simulink model "FaultCheck"  (R2022b)
settings: Solver=FixedStepAuto  StartTime=0.0  StopTime=10  FixedStep=1  RelTol=1e-3
undefined symbols (not defined in the file): C_Flt_IGBTULowerTempConfirmTh_u16, C_Flt_IGBTULowerTempDiagEn_b, C_Flt_IGBTULowerTempErrCode_u16, C_Flt_IGBTULowerTempPowerCoeff, C_Flt_IGBTULowerTempRecoveryTh_u16, C_Flt_IGBTULowerTempRecTh_s32, C_Flt_IGBTULowerTempTrigTh_s32, C_Flt_IGBTUOverTempConfirmTh_u16, C_Flt_IGBTUOverTempDiagEn_b, C_Flt_IGBTUOverTempErrCode_u16, C_Flt_IGBTUOverTempRecoveryTh_u16, C_Flt_IGBTUOverTempRecTh_s32, C_Flt_IGBTUOverTempTrigTh_s32, C_Flt_IGBTVLowerTempConfirmTh_u16, C_Flt_IGBTVLowerTempDiagEn_b, C_Flt_IGBTVLowerTempErrCode_u16, C_Flt_IGBTVLowerTempPowerCoeff, C_Flt_IGBTVLowerTempRecoveryTh_u16, C_Flt_IGBTVLowerTempRecTh_s32, C_Flt_IGBTVLowerTempTrigTh_s32, C_Flt_IGBTVOverTempConfirmTh_u16, C_Flt_IGBTVOverTempDiagEn_b, C_Flt_IGBTVOverTempErrCode_u16, C_Flt_IGBTVOverTempRecoveryTh_u16, C_Flt_IGBTVOverTempRecTh_s32, C_Flt_IGBTVOverTempTrigTh_s32, C_Flt_IGBTWLowerTempConfirmTh_u16, C_Flt_IGBTWLowerTempDiagEn_b, C_Flt_IGBTWLowerTempErrCode_u16, C_Flt_IGBTWLowerTempPowerCoeff, C_Flt_IGBTWLowerTempRecoveryTh_u16, C_Flt_IGBTWLowerTempRecTh_s32, C_Flt_IGBTWLowerTempTrigTh_s32, C_Flt_IGBTWOverTempConfirmTh_u16, C_Flt_IGBTWOverTempDiagEn_b, C_Flt_IGBTWOverTempErrCode_u16, C_Flt_IGBTWOverTempRecoveryTh_u16, C_Flt_IGBTWOverTempRecTh_s32, C_Flt_IGBTWOverTempTrigTh_s32, C_Flt_IuOCConfirmTh_u16, C_Flt_IuOCDiagEn_b, C_Flt_IuOCErrCode_u16, C_Flt_IuOCNegLimit_s32, C_Flt_IuOCPosLimit_s32, C_Flt_IuOCRecoveryTh_u16, C_Flt_IuZeroDriftDiagEn_b, C_Flt_IuZeroDriftErrCode_u16, C_Flt_IvOCConfirmTh_u16, C_Flt_IvOCDiagEn_b, C_Flt_IvOCErrCode_u16, C_Flt_IvOCNegLimit_s32, C_Flt_IvOCPosLimit_s32, C_Flt_IvOCRecoveryTh_u16, C_Flt_IvZeroDriftDiagEn_b, C_Flt_IvZeroDriftErrCode_u16, C_Flt_IwOCConfirmTh_u16, C_Flt_IwOCDiagEn_b, C_Flt_IwOCErrCode_u16, C_Flt_IwOCNegLimit_s32, C_Flt_IwOCPosLimit_s32 ... (+196)
libraries: YS_UserDefined_Library x21, simulink x5
(part 8 of 11)

== system FaultCheck/FaultDiagnose/IGBTTempDiag/IGBTVLowerTempDiag/Diagnose/NormalDiag ==
  IGBTVTemp : Inport
  Parameter : Inport  Port=2
  Action Port : ActionPort  ActionPortLabel=else
  Bus Selector : BusSelector  OutputSignals=IGBTVLowerTempConfirmTh,IGBTVLowerTempRecoveryTh,IGBTVLowerTempTrigTh,IGBTVLowerTempRecTh
  DebounceRecInTwo : YS_UserDefined_Library/Fault/DebounceRecInTwo  SystemSampleTime=-1  VariantActivationTime=update diagram  Latency=0  AutoFrameSizeCalculation=off
      settings: SourceProductName=YS
  Relational Operator : RelationalOperator  Operator=>  OutDataTypeStr=boolean  RndMeth=Simplest  InputSameDT=off
  Relational Operator1 : RelationalOperator  Operator=>  OutDataTypeStr=boolean  RndMeth=Simplest  InputSameDT=off
  Signal Copy : SignalConversion  OverrideOpt=off
  IGBTVLowerTempFltDeb : Outport
  wires:
  Parameter/1 -> Bus Selector/1
  Bus Selector/1 -> DebounceRecInTwo/1  "<IGBTVLowerTempConfirmTh>"
  Bus Selector/2 -> DebounceRecInTwo/2  "<IGBTVLowerTempRecoveryTh>"
  DebounceRecInTwo/1 -> Signal Copy/1  "M_Flt_IGBTVLowerTempFltFlgDeb_b"
  Relational Operator/1 -> DebounceRecInTwo/3  "M_Flt_IGBTVLowerTempFltFlgUnDeb_b"
  Signal Copy/1 -> IGBTVLowerTempFltDeb/1
  Bus Selector/3 -> Relational Operator/1  "<IGBTVLowerTempTrigTh>"
  IGBTVTemp/1 -> Relational Operator1/1, Relational Operator/2
  Bus Selector/4 -> Relational Operator1/2  "<IGBTVLowerTempRecTh>"
  Relational Operator1/1 -> DebounceRecInTwo/4  "M_Flt_IGBTVLowerTempRecFlgUnDeb_b"

== system FaultCheck/FaultDiagnose/IGBTTempDiag/IGBTVLowerTempDiag/FaultLevelDeter/LowerOne ==
  FaultLevel : Inport
  Action Port : ActionPort  ActionPortLabel=else
  IGBTVLowerTempFltLevel : Outport
  wires:
  FaultLevel/1 -> IGBTVLowerTempFltLevel/1

== system FaultCheck/FaultDiagnose/IGBTTempDiag/IGBTVLowerTempDiag/FaultLevelDeter/Normal ==
  Action Port : ActionPort  ActionPortLabel=if(u1 == 0)
  Constant : Constant  Value=C_Flt_LevelZero_u8
  IGBTVLowerTempFltLevel : Outport
  wires:
  Constant/1 -> IGBTVLowerTempFltLevel/1

== system FaultCheck/FaultDiagnose/IGBTTempDiag/IGBTVLowerTempDiag/PowerReductionCoeffDeter/If Action Subsystem ==
  Action Port : ActionPort  ActionPortLabel=if(u1 < 2)
  Constant : Constant  Value=C_Flt_PowerCoeffOne_s32
  Coeff : Outport
  wires:
  Constant/1 -> Coeff/1

== system FaultCheck/FaultDiagnose/IGBTTempDiag/IGBTVLowerTempDiag/PowerReductionCoeffDeter/If Action Subsystem1 ==
  PowerCoeff : Inport
  Action Port : ActionPort  ActionPortLabel=elseif(u1 == 2)
  Coeff : Outport
  wires:
  PowerCoeff/1 -> Coeff/1

== system FaultCheck/FaultDiagnose/IGBTTempDiag/IGBTVLowerTempDiag/PowerReductionCoeffDeter/If Action Subsystem2 ==
  Action Port : ActionPort  ActionPortLabel=else
  Constant : Constant  Value=C_Flt_PowerCoeffZero_s32
  Coeff : Outport
  wires:
  Constant/1 -> Coeff/1

== system FaultCheck/FaultDiagnose/IGBTTempDiag/IGBTVOverTempDiag/Diagnose/Disable ==
  Action Port : ActionPort  ActionPortLabel=if(u1 == 0)
  Constant : Constant  Value=C_Flt_NoErr_b
  IGBTVOverTempFltDeb : Outport
  wires:
  Constant/1 -> IGBTVOverTempFltDeb/1

== system FaultCheck/FaultDiagnose/IGBTTempDiag/IGBTVOverTempDiag/Diagnose/NormalDiag ==
  IGBTVTemp : Inport
  Parameter : Inport  Port=2
  Action Port : ActionPort  ActionPortLabel=else
  Bus Selector : BusSelector  OutputSignals=IGBTVOverTempConfirmTh,IGBTVOverTempRecoveryTh,IGBTVOverTempTrigTh,IGBTVOverTempRecTh
  DebounceRecInTwo : YS_UserDefined_Library/Fault/DebounceRecInTwo  SystemSampleTime=-1  VariantActivationTime=update diagram  Latency=0  AutoFrameSizeCalculation=off
      settings: SourceProductName=YS
  Relational Operator : RelationalOperator  Operator=<  OutDataTypeStr=boolean  RndMeth=Simplest  InputSameDT=off
  Relational Operator1 : RelationalOperator  Operator=<  OutDataTypeStr=boolean  RndMeth=Simplest  InputSameDT=off
  Signal Copy : SignalConversion  OverrideOpt=off
  IGBTVOverTempFltDeb : Outport
  wires:
  Relational Operator1/1 -> DebounceRecInTwo/4  "M_Flt_IGBTVOverTempRecFlgUnDeb_b"
  Bus Selector/4 -> Relational Operator1/2  "<IGBTVOverTempRecTh>"
  IGBTVTemp/1 -> Relational Operator1/1, Relational Operator/2
  Bus Selector/3 -> Relational Operator/1  "<IGBTVOverTempTrigTh>"
  Signal Copy/1 -> IGBTVOverTempFltDeb/1
  Relational Operator/1 -> DebounceRecInTwo/3  "M_Flt_IGBTVOverTempFltFlgUnDeb_b"
  DebounceRecInTwo/1 -> Signal Copy/1  "M_Flt_IGBTVOverTempFltFlgDeb_b"
  Bus Selector/2 -> DebounceRecInTwo/2  "<IGBTVOverTempRecoveryTh>"
  Bus Selector/1 -> DebounceRecInTwo/1  "<IGBTVOverTempConfirmTh>"
  Parameter/1 -> Bus Selector/1

== system FaultCheck/FaultDiagnose/IGBTTempDiag/IGBTVOverTempDiag/FaultLevelDeter/LowerOne ==
  FaultLevel : Inport
  Action Port : ActionPort  ActionPortLabel=else
  IGBTVOverTempFltLevel : Outport
  wires:
  FaultLevel/1 -> IGBTVOverTempFltLevel/1

== system FaultCheck/FaultDiagnose/IGBTTempDiag/IGBTVOverTempDiag/FaultLevelDeter/Normal ==
  Action Port : ActionPort  ActionPortLabel=if(u1 == 0)
  Constant : Constant  Value=C_Flt_LevelZero_u8
  IGBTVOverTempFltLevel : Outport
  wires:
  Constant/1 -> IGBTVOverTempFltLevel/1

== system FaultCheck/FaultDiagnose/IGBTTempDiag/IGBTVOverTempDiag/PowerReductionCoeffDeter/If Action Subsystem ==
  Action Port : ActionPort  ActionPortLabel=if(u1 < 2)
  Constant : Constant  Value=C_Flt_PowerCoeffOne_s32
  Coeff : Outport
  wires:
  Constant/1 -> Coeff/1

== system FaultCheck/FaultDiagnose/IGBTTempDiag/IGBTVOverTempDiag/PowerReductionCoeffDeter/If Action Subsystem1 ==
  PowerCoeff : Inport
  Action Port : ActionPort  ActionPortLabel=elseif(u1 == 2)
  Coeff : Outport
  wires:
  PowerCoeff/1 -> Coeff/1

== system FaultCheck/FaultDiagnose/IGBTTempDiag/IGBTVOverTempDiag/PowerReductionCoeffDeter/If Action Subsystem2 ==
  Action Port : ActionPort  ActionPortLabel=else
  Constant : Constant  Value=C_Flt_PowerCoeffZero_s32
  Coeff : Outport
  wires:
  Constant/1 -> Coeff/1

== system FaultCheck/FaultDiagnose/IGBTTempDiag/IGBTWLowerTempDiag/Diagnose/Disable ==
  Action Port : ActionPort  ActionPortLabel=if(u1 == 0)
  Constant : Constant  Value=C_Flt_NoErr_b
  IGBTWLowerTempFltDeb : Outport
  wires:
  Constant/1 -> IGBTWLowerTempFltDeb/1

== system FaultCheck/FaultDiagnose/IGBTTempDiag/IGBTWLowerTempDiag/Diagnose/NormalDiag ==
  IGBTWTemp : Inport
  Parameter : Inport  Port=2
  Action Port : ActionPort  ActionPortLabel=else
  Bus Selector : BusSelector  OutputSignals=IGBTWLowerTempConfirmTh,IGBTWLowerTempRecoveryTh,IGBTWLowerTempTrigTh,IGBTWLowerTempRecTh
  DebounceRecInTwo : YS_UserDefined_Library/Fault/DebounceRecInTwo  SystemSampleTime=-1  VariantActivationTime=update diagram  Latency=0  AutoFrameSizeCalculation=off
      settings: SourceProductName=YS
  Relational Operator : RelationalOperator  Operator=>  OutDataTypeStr=boolean  RndMeth=Simplest  InputSameDT=off
  Relational Operator1 : RelationalOperator  Operator=>  OutDataTypeStr=boolean  RndMeth=Simplest  InputSameDT=off
  Signal Copy : SignalConversion  OverrideOpt=off
  IGBTWLowerTempFltDeb : Outport
  wires:
  Parameter/1 -> Bus Selector/1
  Bus Selector/1 -> DebounceRecInTwo/1  "<IGBTWLowerTempConfirmTh>"
  Bus Selector/2 -> DebounceRecInTwo/2  "<IGBTWLowerTempRecoveryTh>"
  DebounceRecInTwo/1 -> Signal Copy/1  "M_Flt_IGBTWLowerTempFltFlgDeb_b"
  Relational Operator/1 -> DebounceRecInTwo/3  "M_Flt_IGBTWLowerTempFltFlgUnDeb_b"
  Signal Copy/1 -> IGBTWLowerTempFltDeb/1
  Bus Selector/3 -> Relational Operator/1  "<IGBTWLowerTempTrigTh>"
  IGBTWTemp/1 -> Relational Operator1/1, Relational Operator/2
  Bus Selector/4 -> Relational Operator1/2  "<IGBTWLowerTempRecTh>"
  Relational Operator1/1 -> DebounceRecInTwo/4  "M_Flt_IGBTWLowerTempRecFlgUnDeb_b"

== system FaultCheck/FaultDiagnose/IGBTTempDiag/IGBTWLowerTempDiag/FaultLevelDeter/LowerOne ==
  FaultLevel : Inport
  Action Port : ActionPort  ActionPortLabel=else
  IGBTWLowerTempFltLevel : Outport
  wires:
  FaultLevel/1 -> IGBTWLowerTempFltLevel/1

== system FaultCheck/FaultDiagnose/IGBTTempDiag/IGBTWLowerTempDiag/FaultLevelDeter/Normal ==
  Action Port : ActionPort  ActionPortLabel=if(u1 == 0)
  Constant : Constant  Value=C_Flt_LevelZero_u8
  IGBTWLowerTempFltLevel : Outport
  wires:
  Constant/1 -> IGBTWLowerTempFltLevel/1

== system FaultCheck/FaultDiagnose/IGBTTempDiag/IGBTWLowerTempDiag/PowerReductionCoeffDeter/If Action Subsystem ==
  Action Port : ActionPort  ActionPortLabel=if(u1 < 2)
  Constant : Constant  Value=C_Flt_PowerCoeffOne_s32
  Coeff : Outport
  wires:
  Constant/1 -> Coeff/1

== system FaultCheck/FaultDiagnose/IGBTTempDiag/IGBTWLowerTempDiag/PowerReductionCoeffDeter/If Action Subsystem1 ==
  PowerCoeff : Inport
  Action Port : ActionPort  ActionPortLabel=elseif(u1 == 2)
  Coeff : Outport
  wires:
  PowerCoeff/1 -> Coeff/1

== system FaultCheck/FaultDiagnose/IGBTTempDiag/IGBTWLowerTempDiag/PowerReductionCoeffDeter/If Action Subsystem2 ==
  Action Port : ActionPort  ActionPortLabel=else
  Constant : Constant  Value=C_Flt_PowerCoeffZero_s32
  Coeff : Outport
  wires:
  Constant/1 -> Coeff/1

== system FaultCheck/FaultDiagnose/IGBTTempDiag/IGBTWOverTempDiag/Diagnose/Disable ==
  Action Port : ActionPort  ActionPortLabel=if(u1 == 0)
  Constant : Constant  Value=C_Flt_NoErr_b
  IGBTWOverTempFltDeb : Outport
  wires:
  Constant/1 -> IGBTWOverTempFltDeb/1

== system FaultCheck/FaultDiagnose/IGBTTempDiag/IGBTWOverTempDiag/Diagnose/NormalDiag ==
  IGBTWTemp : Inport
  Parameter : Inport  Port=2
  Action Port : ActionPort  ActionPortLabel=else
  Bus Selector : BusSelector  OutputSignals=IGBTWOverTempConfirmTh,IGBTWOverTempRecoveryTh,IGBTWOverTempTrigTh,IGBTWOverTempRecTh
  DebounceRecInTwo : YS_UserDefined_Library/Fault/DebounceRecInTwo  SystemSampleTime=-1  VariantActivationTime=update diagram  Latency=0  AutoFrameSizeCalculation=off
      settings: SourceProductName=YS
  Relational Operator : RelationalOperator  Operator=<  OutDataTypeStr=boolean  RndMeth=Simplest  InputSameDT=off
  Relational Operator1 : RelationalOperator  Operator=<  OutDataTypeStr=boolean  RndMeth=Simplest  InputSameDT=off
  Signal Copy : SignalConversion  OverrideOpt=off
  IGBTWOverTempFltDeb : Outport
  wires:
  Parameter/1 -> Bus Selector/1
  Bus Selector/1 -> DebounceRecInTwo/1  "<IGBTWOverTempConfirmTh>"
  Bus Selector/2 -> DebounceRecInTwo/2  "<IGBTWOverTempRecoveryTh>"
  DebounceRecInTwo/1 -> Signal Copy/1  "M_Flt_IGBTWOverTempFltFlgDeb_b"
  Relational Operator/1 -> DebounceRecInTwo/3  "M_Flt_IGBTWOverTempFltFlgUnDeb_b"
  Signal Copy/1 -> IGBTWOverTempFltDeb/1
  Bus Selector/3 -> Relational Operator/1  "<IGBTWOverTempTrigTh>"
  IGBTWTemp/1 -> Relational Operator1/1, Relational Operator/2
  Bus Selector/4 -> Relational Operator1/2  "<IGBTWOverTempRecTh>"
  Relational Operator1/1 -> DebounceRecInTwo/4  "M_Flt_IGBTWOverTempRecFlgUnDeb_b"

== system FaultCheck/FaultDiagnose/IGBTTempDiag/IGBTWOverTempDiag/FaultLevelDeter/LowerOne ==
  FaultLevel : Inport
  Action Port : ActionPort  ActionPortLabel=else
  IGBTWOverTempFltLevel : Outport
  wires:
  FaultLevel/1 -> IGBTWOverTempFltLevel/1

== system FaultCheck/FaultDiagnose/IGBTTempDiag/IGBTWOverTempDiag/FaultLevelDeter/Normal ==
  Action Port : ActionPort  ActionPortLabel=if(u1 == 0)
  Constant : Constant  Value=C_Flt_LevelZero_u8
  IGBTWOverTempFltLevel : Outport
  wires:
  Constant/1 -> IGBTWOverTempFltLevel/1

== system FaultCheck/FaultDiagnose/IGBTTempDiag/IGBTWOverTempDiag/PowerReductionCoeffDeter/If Action Subsystem ==
  Action Port : ActionPort  ActionPortLabel=if(u1 < 2)
  Constant : Constant  Value=C_Flt_PowerCoeffOne_s32
  Coeff : Outport
  wires:
  Constant/1 -> Coeff/1

== system FaultCheck/FaultDiagnose/IGBTTempDiag/IGBTWOverTempDiag/PowerReductionCoeffDeter/If Action Subsystem1 ==
  PowerCoeff : Inport
  Action Port : ActionPort  ActionPortLabel=elseif(u1 == 2)
  Coeff : Outport
  wires:
  PowerCoeff/1 -> Coeff/1

== system FaultCheck/FaultDiagnose/IGBTTempDiag/IGBTWOverTempDiag/PowerReductionCoeffDeter/If Action Subsystem2 ==
  Action Port : ActionPort  ActionPortLabel=else
  Constant : Constant  Value=C_Flt_PowerCoeffZero_s32
  Coeff : Outport
  wires:
  Constant/1 -> Coeff/1

== system FaultCheck/FaultDiagnose/MotorSpdFltDiag/MotorOverSpdOneNegDiag/Diagnose/Disable ==
  Action Port : ActionPort  ActionPortLabel=if(u1 == 0)
  Constant : Constant  Value=C_Flt_NoErr_b
  MotorOverSpdOneNegFltDeb : Outport
  wires:
  Constant/1 -> MotorOverSpdOneNegFltDeb/1

== system FaultCheck/FaultDiagnose/MotorSpdFltDiag/MotorOverSpdOneNegDiag/Diagnose/NormalDiag ==
  MotorSpd : Inport
  Parameter : Inport  Port=2
  Action Port : ActionPort  ActionPortLabel=else
  Bus Selector : BusSelector  OutputSignals=MotorOverSpdOneNegConfirmTh,MotorOverSpdOneNegRecoveryTh,MotorOverSpdOneNegTrigTh,MotorOverSpdOneNegRecTh
  DebounceRecInTwo : YS_UserDefined_Library/Fault/DebounceRecInTwo  SystemSampleTime=-1  VariantActivationTime=update diagram  Latency=0  AutoFrameSizeCalculation=off
      settings: SourceProductName=YS
  Relational Operator : RelationalOperator  Operator=>  OutDataTypeStr=boolean  RndMeth=Simplest  InputSameDT=off
  Relational Operator1 : RelationalOperator  Operator=>  OutDataTypeStr=boolean  RndMeth=Simplest  InputSameDT=off
  Signal Copy : SignalConversion  OverrideOpt=off
  MotorOverSpdOneNegFltDeb : Outport
  wires:
  Parameter/1 -> Bus Selector/1
  Bus Selector/1 -> DebounceRecInTwo/1  "<MotorOverSpdOneNegConfirmTh>"
  Bus Selector/2 -> DebounceRecInTwo/2  "<MotorOverSpdOneNegRecoveryTh>"
  DebounceRecInTwo/1 -> Signal Copy/1  "M_Flt_MotorOverSpdOneNegFltFlgDeb_b"
  Relational Operator/1 -> DebounceRecInTwo/3  "M_Flt_MotorOverSpdOneNegFltFlgUnDeb_b"
  Signal Copy/1 -> MotorOverSpdOneNegFltDeb/1
  Bus Selector/3 -> Relational Operator/1  "<MotorOverSpdOneNegTrigTh>"
  MotorSpd/1 -> Relational Operator1/1, Relational Operator/2
  Bus Selector/4 -> Relational Operator1/2  "<MotorOverSpdOneNegRecTh>"
  Relational Operator1/1 -> DebounceRecInTwo/4  "M_Flt_MotorOverSpdOneNegRecFlgUnDeb_b"

== system FaultCheck/FaultDiagnose/MotorSpdFltDiag/MotorOverSpdOneNegDiag/FaultLevelDeter/LowerOne ==
  FaultLevel : Inport
  Action Port : ActionPort  ActionPortLabel=else
  MotorOverSpdOneNegFltLevel : Outport
  wires:
  FaultLevel/1 -> MotorOverSpdOneNegFltLevel/1

== system FaultCheck/FaultDiagnose/MotorSpdFltDiag/MotorOverSpdOneNegDiag/FaultLevelDeter/Normal ==
  Action Port : ActionPort  ActionPortLabel=if(u1 == 0)
  Constant : Constant  Value=C_Flt_LevelZero_u8
  MotorOverSpdOneNegFltLevel : Outport
  wires:
  Constant/1 -> MotorOverSpdOneNegFltLevel/1

== system FaultCheck/FaultDiagnose/MotorSpdFltDiag/MotorOverSpdOneNegDiag/PowerReductionCoeffDeter/If Action Subsystem ==
  Action Port : ActionPort  ActionPortLabel=if(u1 < 2)
  Constant : Constant  Value=C_Flt_PowerCoeffOne_s32
  Coeff : Outport
  wires:
  Constant/1 -> Coeff/1

== system FaultCheck/FaultDiagnose/MotorSpdFltDiag/MotorOverSpdOneNegDiag/PowerReductionCoeffDeter/If Action Subsystem1 ==
  PowerCoeff : Inport
  Action Port : ActionPort  ActionPortLabel=elseif(u1 == 2)
  Coeff : Outport
  wires:
  PowerCoeff/1 -> Coeff/1

== system FaultCheck/FaultDiagnose/MotorSpdFltDiag/MotorOverSpdOneNegDiag/PowerReductionCoeffDeter/If Action Subsystem2 ==
  Action Port : ActionPort  ActionPortLabel=else
  Constant : Constant  Value=C_Flt_PowerCoeffZero_s32
  Coeff : Outport
  wires:
  Constant/1 -> Coeff/1

== system FaultCheck/FaultDiagnose/MotorSpdFltDiag/MotorOverSpdOnePosDiag/Diagnose/Disable ==
  Action Port : ActionPort  ActionPortLabel=if(u1 == 0)
  Constant : Constant  Value=C_Flt_NoErr_b
  MotorOverSpdOnePosFltDeb : Outport
  wires:
  Constant/1 -> MotorOverSpdOnePosFltDeb/1

== system FaultCheck/FaultDiagnose/MotorSpdFltDiag/MotorOverSpdOnePosDiag/Diagnose/NormalDiag ==
  MotorSpd : Inport
  Parameter : Inport  Port=2
  Action Port : ActionPort  ActionPortLabel=else
  Bus Selector : BusSelector  OutputSignals=MotorOverSpdOnePosConfirmTh,MotorOverSpdOnePosRecoveryTh,MotorOverSpdOnePosTrigTh,MotorOverSpdOnePosRecTh
  DebounceRecInTwo : YS_UserDefined_Library/Fault/DebounceRecInTwo  SystemSampleTime=-1  VariantActivationTime=update diagram  Latency=0  AutoFrameSizeCalculation=off
      settings: SourceProductName=YS
  Relational Operator : RelationalOperator  Operator=<  OutDataTypeStr=boolean  RndMeth=Simplest  InputSameDT=off
  Relational Operator1 : RelationalOperator  Operator=<  OutDataTypeStr=boolean  RndMeth=Simplest  InputSameDT=off
  Signal Copy : SignalConversion  OverrideOpt=off
  MotorOverSpdOnePosFltDeb : Outport
  wires:
  Parameter/1 -> Bus Selector/1
  Bus Selector/1 -> DebounceRecInTwo/1  "<MotorOverSpdOnePosConfirmTh>"
  Bus Selector/2 -> DebounceRecInTwo/2  "<MotorOverSpdOnePosRecoveryTh>"
  DebounceRecInTwo/1 -> Signal Copy/1  "M_Flt_MotorOverSpdOnePosFltFlgDeb_b"
  Relational Operator/1 -> DebounceRecInTwo/3  "M_Flt_MotorOverSpdOnePosFltFlgUnDeb_b"
  Signal Copy/1 -> MotorOverSpdOnePosFltDeb/1
  Bus Selector/3 -> Relational Operator/1  "<MotorOverSpdOnePosTrigTh>"
  MotorSpd/1 -> Relational Operator1/1, Relational Operator/2
  Bus Selector/4 -> Relational Operator1/2  "<MotorOverSpdOnePosRecTh>"
  Relational Operator1/1 -> DebounceRecInTwo/4  "M_Flt_MotorOverSpdOnePosRecFlgUnDeb_b"

== system FaultCheck/FaultDiagnose/MotorSpdFltDiag/MotorOverSpdOnePosDiag/FaultLevelDeter/LowerOne ==
  FaultLevel : Inport
  Action Port : ActionPort  ActionPortLabel=else
  MotorOverSpdOnePosFltLevel : Outport
  wires:
  FaultLevel/1 -> MotorOverSpdOnePosFltLevel/1

== system FaultCheck/FaultDiagnose/MotorSpdFltDiag/MotorOverSpdOnePosDiag/FaultLevelDeter/Normal ==
  Action Port : ActionPort  ActionPortLabel=if(u1 == 0)
  Constant : Constant  Value=C_Flt_LevelZero_u8
  MotorOverSpdOnePosFltLevel : Outport
  wires:
  Constant/1 -> MotorOverSpdOnePosFltLevel/1

== system FaultCheck/FaultDiagnose/MotorSpdFltDiag/MotorOverSpdOnePosDiag/PowerReductionCoeffDeter/If Action Subsystem ==
  Action Port : ActionPort  ActionPortLabel=if(u1 < 2)
  Constant : Constant  Value=C_Flt_PowerCoeffOne_s32
  Coeff : Outport
  wires:
  Constant/1 -> Coeff/1

== system FaultCheck/FaultDiagnose/MotorSpdFltDiag/MotorOverSpdOnePosDiag/PowerReductionCoeffDeter/If Action Subsystem1 ==
  PowerCoeff : Inport
  Action Port : ActionPort  ActionPortLabel=elseif(u1 == 2)
  Coeff : Outport
  wires:
  PowerCoeff/1 -> Coeff/1

== system FaultCheck/FaultDiagnose/MotorSpdFltDiag/MotorOverSpdOnePosDiag/PowerReductionCoeffDeter/If Action Subsystem2 ==
  Action Port : ActionPort  ActionPortLabel=else
  Constant : Constant  Value=C_Flt_PowerCoeffZero_s32
  Coeff : Outport
  wires:
  Constant/1 -> Coeff/1

== system FaultCheck/FaultDiagnose/MotorSpdFltDiag/MotorOverSpdTwoNegDiag/Diagnose/Disable ==
  Action Port : ActionPort  ActionPortLabel=if(u1 == 0)
  Constant : Constant  Value=C_Flt_NoErr_b
  MotorOverSpdTwoNegFltDeb : Outport
  wires:
  Constant/1 -> MotorOverSpdTwoNegFltDeb/1

== system FaultCheck/FaultDiagnose/MotorSpdFltDiag/MotorOverSpdTwoNegDiag/Diagnose/NormalDiag ==
  PCBTemp : Inport
  Parameter : Inport  Port=2
  Action Port : ActionPort  ActionPortLabel=else
  Bus Selector : BusSelector  OutputSignals=MotorOverSpdTwoNegConfirmTh,MotorOverSpdTwoNegRecoveryTh,MotorOverSpdTwoNegTrigTh,MotorOverSpdTwoNegRecTh
  DebounceRecInTwo : YS_UserDefined_Library/Fault/DebounceRecInTwo  SystemSampleTime=-1  VariantActivationTime=update diagram  Latency=0  AutoFrameSizeCalculation=off
      settings: SourceProductName=YS
  Relational Operator : RelationalOperator  Operator=>  OutDataTypeStr=boolean  RndMeth=Simplest  InputSameDT=off
  Relational Operator1 : RelationalOperator  Operator=>  OutDataTypeStr=boolean  RndMeth=Simplest  InputSameDT=off
  Signal Copy : SignalConversion  OverrideOpt=off
  MotorOverSpdTwoNegFltDeb : Outport
  wires:
  Relational Operator1/1 -> DebounceRecInTwo/4  "M_Flt_MotorOverSpdTwoNegRecFlgUnDeb_b"
  Bus Selector/4 -> Relational Operator1/2  "<MotorOverSpdTwoNegRecTh>"
  PCBTemp/1 -> Relational Operator1/1, Relational Operator/2
  Bus Selector/3 -> Relational Operator/1  "<MotorOverSpdTwoNegTrigTh>"
  Signal Copy/1 -> MotorOverSpdTwoNegFltDeb/1
  Relational Operator/1 -> DebounceRecInTwo/3  "M_Flt_MotorOverSpdTwoNegFltFlgUnDeb_b"
  DebounceRecInTwo/1 -> Signal Copy/1  "M_Flt_MotorOverSpdTwoNegFltFlgDeb_b"
  Bus Selector/2 -> DebounceRecInTwo/2  "<MotorOverSpdTwoNegRecoveryTh>"
  Bus Selector/1 -> DebounceRecInTwo/1  "<MotorOverSpdTwoNegConfirmTh>"
  Parameter/1 -> Bus Selector/1

== system FaultCheck/FaultDiagnose/MotorSpdFltDiag/MotorOverSpdTwoNegDiag/FaultLevelDeter/LowerOne ==
  FaultLevel : Inport
  Action Port : ActionPort  ActionPortLabel=else
  MotorOverSpdTwoNegFltLevel : Outport
  wires:
  FaultLevel/1 -> MotorOverSpdTwoNegFltLevel/1

== system FaultCheck/FaultDiagnose/MotorSpdFltDiag/MotorOverSpdTwoNegDiag/FaultLevelDeter/Normal ==
  Action Port : ActionPort  ActionPortLabel=if(u1 == 0)
  Constant : Constant  Value=C_Flt_LevelZero_u8
  MotorOverSpdTwoNegFltLevel : Outport
  wires:
  Constant/1 -> MotorOverSpdTwoNegFltLevel/1

== system FaultCheck/FaultDiagnose/MotorSpdFltDiag/MotorOverSpdTwoNegDiag/PowerReductionCoeffDeter/If Action Subsystem ==
  Action Port : ActionPort  ActionPortLabel=if(u1 < 2)
  Constant : Constant  Value=C_Flt_PowerCoeffOne_s32
  Coeff : Outport
  wires:
  Constant/1 -> Coeff/1

== system FaultCheck/FaultDiagnose/MotorSpdFltDiag/MotorOverSpdTwoNegDiag/PowerReductionCoeffDeter/If Action Subsystem1 ==
  PowerCoeff : Inport
  Action Port : ActionPort  ActionPortLabel=elseif(u1 == 2)
  Coeff : Outport
  wires:
  PowerCoeff/1 -> Coeff/1

== system FaultCheck/FaultDiagnose/MotorSpdFltDiag/MotorOverSpdTwoNegDiag/PowerReductionCoeffDeter/If Action Subsystem2 ==
  Action Port : ActionPort  ActionPortLabel=else
  Constant : Constant  Value=C_Flt_PowerCoeffZero_s32
  Coeff : Outport
  wires:
  Constant/1 -> Coeff/1

== system FaultCheck/FaultDiagnose/MotorSpdFltDiag/MotorOverSpdTwoPosDiag/Diagnose/Disable ==
  Action Port : ActionPort  ActionPortLabel=if(u1 == 0)
  Constant : Constant  Value=C_Flt_NoErr_b
  MotorOverSpdTwoPosFltDeb : Outport
  wires:
  Constant/1 -> MotorOverSpdTwoPosFltDeb/1

== system FaultCheck/FaultDiagnose/MotorSpdFltDiag/MotorOverSpdTwoPosDiag/Diagnose/NormalDiag ==
  MotorSpd : Inport
  Parameter : Inport  Port=2
  Action Port : ActionPort  ActionPortLabel=else
  Bus Selector : BusSelector  OutputSignals=MotorOverSpdTwoPosConfirmTh,MotorOverSpdTwoPosRecoveryTh,MotorOverSpdTwoPosTrigTh,MotorOverSpdTwoPosRecTh
  DebounceRecInTwo : YS_UserDefined_Library/Fault/DebounceRecInTwo  SystemSampleTime=-1  VariantActivationTime=update diagram  Latency=0  AutoFrameSizeCalculation=off
      settings: SourceProductName=YS
  Relational Operator : RelationalOperator  Operator=<  OutDataTypeStr=boolean  RndMeth=Simplest  InputSameDT=off
  Relational Operator1 : RelationalOperator  Operator=<  OutDataTypeStr=boolean  RndMeth=Simplest  InputSameDT=off
  Signal Copy : SignalConversion  OverrideOpt=off
  MotorOverSpdTwoPosFltDeb : Outport
  wires:
  Relational Operator1/1 -> DebounceRecInTwo/4  "M_Flt_MotorOverSpdTwoPosRecFlgUnDeb_b"
  Bus Selector/4 -> Relational Operator1/2  "<MotorOverSpdTwoPosRecTh>"
  MotorSpd/1 -> Relational Operator1/1, Relational Operator/2
  Bus Selector/3 -> Relational Operator/1  "<MotorOverSpdTwoPosTrigTh>"
  Signal Copy/1 -> MotorOverSpdTwoPosFltDeb/1
  Relational Operator/1 -> DebounceRecInTwo/3  "M_Flt_MotorOverSpdTwoPosFltFlgUnDeb_b"
  DebounceRecInTwo/1 -> Signal Copy/1  "M_Flt_MotorOverSpdTwoPosFltFlgDeb_b"
  Bus Selector/2 -> DebounceRecInTwo/2  "<MotorOverSpdTwoPosRecoveryTh>"
  Bus Selector/1 -> DebounceRecInTwo/1  "<MotorOverSpdTwoPosConfirmTh>"
  Parameter/1 -> Bus Selector/1

== system FaultCheck/FaultDiagnose/MotorSpdFltDiag/MotorOverSpdTwoPosDiag/FaultLevelDeter/LowerOne ==
  FaultLevel : Inport
  Action Port : ActionPort  ActionPortLabel=else
  MotorOverSpdTwoPosFltLevel : Outport
  wires:
  FaultLevel/1 -> MotorOverSpdTwoPosFltLevel/1

== system FaultCheck/FaultDiagnose/MotorSpdFltDiag/MotorOverSpdTwoPosDiag/FaultLevelDeter/Normal ==
  Action Port : ActionPort  ActionPortLabel=if(u1 == 0)
  Constant : Constant  Value=C_Flt_LevelZero_u8
  MotorOverSpdTwoPosFltLevel : Outport
  wires:
  Constant/1 -> MotorOverSpdTwoPosFltLevel/1

== system FaultCheck/FaultDiagnose/MotorSpdFltDiag/MotorOverSpdTwoPosDiag/PowerReductionCoeffDeter/If Action Subsystem ==
  Action Port : ActionPort  ActionPortLabel=if(u1 < 2)
  Constant : Constant  Value=C_Flt_PowerCoeffOne_s32
  Coeff : Outport
  wires:
  Constant/1 -> Coeff/1

== system FaultCheck/FaultDiagnose/MotorSpdFltDiag/MotorOverSpdTwoPosDiag/PowerReductionCoeffDeter/If Action Subsystem1 ==
  PowerCoeff : Inport
  Action Port : ActionPort  ActionPortLabel=elseif(u1 == 2)
  Coeff : Outport
  wires:
  PowerCoeff/1 -> Coeff/1

== system FaultCheck/FaultDiagnose/MotorSpdFltDiag/MotorOverSpdTwoPosDiag/PowerReductionCoeffDeter/If Action Subsystem2 ==
  Action Port : ActionPort  ActionPortLabel=else
  Constant : Constant  Value=C_Flt_PowerCoeffZero_s32
  Coeff : Outport
  wires:
  Constant/1 -> Coeff/1

== system FaultCheck/FaultDiagnose/MotorTempDiag/MotorLowerTempDiag/Diagnose/Disable ==
  Action Port : ActionPort  ActionPortLabel=if(u1 == 0)
  Constant : Constant  Value=C_Flt_NoErr_b
  MotorLowerTempFltDeb : Outport
  wires:
  Constant/1 -> MotorLowerTempFltDeb/1

== system FaultCheck/FaultDiagnose/MotorTempDiag/MotorLowerTempDiag/Diagnose/NormalDiag ==
  MotorTemp : Inport
  Parameter : Inport  Port=2
  Action Port : ActionPort  ActionPortLabel=else
  Bus Selector : BusSelector  OutputSignals=MotorLowerTempConfirmTh,MotorLowerTempRecoveryTh,MotorLowerTempTrigTh,MotorLowerTempRecTh
  DebounceRecInTwo : YS_UserDefined_Library/Fault/DebounceRecInTwo  SystemSampleTime=-1  VariantActivationTime=update diagram  Latency=0  AutoFrameSizeCalculation=off
      settings: SourceProductName=YS
  Relational Operator : RelationalOperator  Operator=>  OutDataTypeStr=boolean  RndMeth=Simplest  InputSameDT=off
  Relational Operator1 : RelationalOperator  Operator=>  OutDataTypeStr=boolean  RndMeth=Simplest  InputSameDT=off
  Signal Copy : SignalConversion  OverrideOpt=off
  MotorLowerTempFltDeb : Outport
  wires:
  Relational Operator1/1 -> DebounceRecInTwo/4  "M_Flt_MotorLowerTempRecFlgUnDeb_b"
  Bus Selector/4 -> Relational Operator1/2  "<MotorLowerTempRecTh>"
  MotorTemp/1 -> Relational Operator/2, Relational Operator1/1
  Bus Selector/3 -> Relational Operator/1  "<MotorLowerTempTrigTh>"
  Signal Copy/1 -> MotorLowerTempFltDeb/1
  Relational Operator/1 -> DebounceRecInTwo/3  "M_Flt_MotorLowerTempFltFlgUnDeb_b"
  DebounceRecInTwo/1 -> Signal Copy/1  "M_Flt_MotorLowerTempFltFlgDeb_b"
  Bus Selector/2 -> DebounceRecInTwo/2  "<MotorLowerTempRecoveryTh>"
  Bus Selector/1 -> DebounceRecInTwo/1  "<MotorLowerTempConfirmTh>"
  Parameter/1 -> Bus Selector/1

== system FaultCheck/FaultDiagnose/MotorTempDiag/MotorLowerTempDiag/FaultLevelDeter/LowerOne ==
  FaultLevel : Inport
  Action Port : ActionPort  ActionPortLabel=else
  MotorLowerTempFltLevel : Outport
  wires:
  FaultLevel/1 -> MotorLowerTempFltLevel/1

== system FaultCheck/FaultDiagnose/MotorTempDiag/MotorLowerTempDiag/FaultLevelDeter/Normal ==
  Action Port : ActionPort  ActionPortLabel=if(u1 == 0)
  Constant : Constant  Value=C_Flt_LevelZero_u8
  MotorLowerTempFltLevel : Outport
  wires:
  Constant/1 -> MotorLowerTempFltLevel/1

== system FaultCheck/FaultDiagnose/MotorTempDiag/MotorLowerTempDiag/PowerReductionCoeffDeter/If Action Subsystem ==
  Action Port : ActionPort  ActionPortLabel=if(u1 < 2)
  Constant : Constant  Value=C_Flt_PowerCoeffOne_s32
  Coeff : Outport
  wires:
  Constant/1 -> Coeff/1

== system FaultCheck/FaultDiagnose/MotorTempDiag/MotorLowerTempDiag/PowerReductionCoeffDeter/If Action Subsystem1 ==
  PowerCoeff : Inport
  Action Port : ActionPort  ActionPortLabel=elseif(u1 == 2)
  Coeff : Outport
  wires:
  PowerCoeff/1 -> Coeff/1

== system FaultCheck/FaultDiagnose/MotorTempDiag/MotorLowerTempDiag/PowerReductionCoeffDeter/If Action Subsystem2 ==
  Action Port : ActionPort  ActionPortLabel=else
  Constant : Constant  Value=C_Flt_PowerCoeffZero_s32
  Coeff : Outport
  wires:
  Constant/1 -> Coeff/1

== system FaultCheck/FaultDiagnose/MotorTempDiag/MotorOverTempDiag/Diagnose/Disable ==
  Action Port : ActionPort  ActionPortLabel=if(u1 == 0)
  Constant : Constant  Value=C_Flt_NoErr_b
  MotorOverTempFltDeb : Outport
  wires:
  Constant/1 -> MotorOverTempFltDeb/1

== system FaultCheck/FaultDiagnose/MotorTempDiag/MotorOverTempDiag/Diagnose/NormalDiag ==
  MotorTemp : Inport
  Parameter : Inport  Port=2
  Action Port : ActionPort  ActionPortLabel=else
  Bus Selector : BusSelector  OutputSignals=MotorOverTempConfirmTh,MotorOverTempRecoveryTh,MotorOverTempTrigTh,MotorOverTempRecTh
  DebounceRecInTwo : YS_UserDefined_Library/Fault/DebounceRecInTwo  SystemSampleTime=-1  VariantActivationTime=update diagram  Latency=0  AutoFrameSizeCalculation=off
      settings: SourceProductName=YS
  Relational Operator : RelationalOperator  Operator=<  OutDataTypeStr=boolean  RndMeth=Simplest  InputSameDT=off
  Relational Operator1 : RelationalOperator  Operator=<  OutDataTypeStr=boolean  RndMeth=Simplest  InputSameDT=off
  Signal Copy : SignalConversion  OverrideOpt=off
  MotorOverTempFltDeb : Outport
  wires:
  Parameter/1 -> Bus Selector/1
  Bus Selector/1 -> DebounceRecInTwo/1  "<MotorOverTempConfirmTh>"
  Bus Selector/2 -> DebounceRecInTwo/2  "<MotorOverTempRecoveryTh>"
  DebounceRecInTwo/1 -> Signal Copy/1  "M_Flt_MotorOverTempFltFlgDeb_b"
  Relational Operator/1 -> DebounceRecInTwo/3  "M_Flt_MotorOverTempFltFlgUnDeb_b"
  Signal Copy/1 -> MotorOverTempFltDeb/1
  Bus Selector/3 -> Relational Operator/1  "<MotorOverTempTrigTh>"
  MotorTemp/1 -> Relational Operator1/1, Relational Operator/2
  Bus Selector/4 -> Relational Operator1/2  "<MotorOverTempRecTh>"
  Relational Operator1/1 -> DebounceRecInTwo/4  "M_Flt_MotorOverTempRecFlgUnDeb_b"

== system FaultCheck/FaultDiagnose/MotorTempDiag/MotorOverTempDiag/FaultLevelDeter/LowerOne ==
  FaultLevel : Inport
  Action Port : ActionPort  ActionPortLabel=else
  MotorOverTempFltLevel : Outport
  wires:
  FaultLevel/1 -> MotorOverTempFltLevel/1

== system FaultCheck/FaultDiagnose/MotorTempDiag/MotorOverTempDiag/FaultLevelDeter/Normal ==
  Action Port : ActionPort  ActionPortLabel=if(u1 == 0)
  Constant : Constant  Value=C_Flt_LevelZero_u8
  MotorOverTempFltLevel : Outport
  wires:
  Constant/1 -> MotorOverTempFltLevel/1

== system FaultCheck/FaultDiagnose/MotorTempDiag/MotorOverTempDiag/PowerReductionCoeffDeter/If Action Subsystem ==
  Action Port : ActionPort  ActionPortLabel=if(u1 < 2)
  Constant : Constant  Value=C_Flt_PowerCoeffOne_s32
  Coeff : Outport
  wires:
  Constant/1 -> Coeff/1

== system FaultCheck/FaultDiagnose/MotorTempDiag/MotorOverTempDiag/PowerReductionCoeffDeter/If Action Subsystem1 ==
  PowerCoeff : Inport
  Action Port : ActionPort  ActionPortLabel=elseif(u1 == 2)
  Coeff : Outport
  wires:
  PowerCoeff/1 -> Coeff/1

== system FaultCheck/FaultDiagnose/MotorTempDiag/MotorOverTempDiag/PowerReductionCoeffDeter/If Action Subsystem2 ==
  Action Port : ActionPort  ActionPortLabel=else
  Constant : Constant  Value=C_Flt_PowerCoeffZero_s32
  Coeff : Outport
  wires:
  Constant/1 -> Coeff/1

== system FaultCheck/FaultDiagnose/PCBTempDiag/PCBLowerTempDiag/Diagnose/Disable ==
  Action Port : ActionPort  ActionPortLabel=if(u1 == 0)
  Constant : Constant  Value=C_Flt_NoErr_b
  PCBLowerTempFltDeb : Outport
  wires:
  Constant/1 -> PCBLowerTempFltDeb/1

== system FaultCheck/FaultDiagnose/PCBTempDiag/PCBLowerTempDiag/Diagnose/NormalDiag ==
  PCBTemp : Inport
  Parameter : Inport  Port=2
  Action Port : ActionPort  ActionPortLabel=else
  Bus Selector : BusSelector  OutputSignals=PCBLowerTempConfirmTh,PCBLowerTempRecoveryTh,PCBLowerTempTrigTh,PCBLowerTempRecTh
  DebounceRecInTwo : YS_UserDefined_Library/Fault/DebounceRecInTwo  SystemSampleTime=-1  VariantActivationTime=update diagram  Latency=0  AutoFrameSizeCalculation=off
      settings: SourceProductName=YS
  Relational Operator : RelationalOperator  Operator=>  OutDataTypeStr=boolean  RndMeth=Simplest  InputSameDT=off
  Relational Operator1 : RelationalOperator  Operator=>  OutDataTypeStr=boolean  RndMeth=Simplest  InputSameDT=off
  Signal Copy : SignalConversion  OverrideOpt=off
  PCBLowerTempFltDeb : Outport
  wires:
  Relational Operator1/1 -> DebounceRecInTwo/4  "M_Flt_PCBLowerTempRecFlgUnDeb_b"
  Bus Selector/4 -> Relational Operator1/2  "<PCBLowerTempRecTh>"
  PCBTemp/1 -> Relational Operator1/1, Relational Operator/2
  Bus Selector/3 -> Relational Operator/1  "<PCBLowerTempTrigTh>"
  Signal Copy/1 -> PCBLowerTempFltDeb/1
  Relational Operator/1 -> DebounceRecInTwo/3  "M_Flt_PCBLowerTempFltFlgUnDeb_b"
  DebounceRecInTwo/1 -> Signal Copy/1  "M_Flt_PCBLowerTempFltFlgDeb_b"
  Bus Selector/2 -> DebounceRecInTwo/2  "<PCBLowerTempRecoveryTh>"
  Bus Selector/1 -> DebounceRecInTwo/1  "<PCBLowerTempConfirmTh>"
  Parameter/1 -> Bus Selector/1

== system FaultCheck/FaultDiagnose/PCBTempDiag/PCBLowerTempDiag/FaultLevelDeter/LowerOne ==
  FaultLevel : Inport
  Action Port : ActionPort  ActionPortLabel=else
  PCBLowerTempFltLevel : Outport
  wires:
  FaultLevel/1 -> PCBLowerTempFltLevel/1

== system FaultCheck/FaultDiagnose/PCBTempDiag/PCBLowerTempDiag/FaultLevelDeter/Normal ==
  Action Port : ActionPort  ActionPortLabel=if(u1 == 0)
  Constant : Constant  Value=C_Flt_LevelZero_u8
  PCBLowerTempFltLevel : Outport
  wires:
  Constant/1 -> PCBLowerTempFltLevel/1

== system FaultCheck/FaultDiagnose/PCBTempDiag/PCBLowerTempDiag/PowerReductionCoeffDeter/If Action Subsystem ==
  Action Port : ActionPort  ActionPortLabel=if(u1 < 2)
  Constant : Constant  Value=C_Flt_PowerCoeffOne_s32
  Coeff : Outport
  wires:
  Constant/1 -> Coeff/1

== system FaultCheck/FaultDiagnose/PCBTempDiag/PCBLowerTempDiag/PowerReductionCoeffDeter/If Action Subsystem1 ==
  PowerCoeff : Inport
  Action Port : ActionPort  ActionPortLabel=elseif(u1 == 2)
  Coeff : Outport
  wires:
  PowerCoeff/1 -> Coeff/1

== system FaultCheck/FaultDiagnose/PCBTempDiag/PCBLowerTempDiag/PowerReductionCoeffDeter/If Action Subsystem2 ==
  Action Port : ActionPort  ActionPortLabel=else
  Constant : Constant  Value=C_Flt_PowerCoeffZero_s32
  Coeff : Outport
  wires:
  Constant/1 -> Coeff/1

== system FaultCheck/FaultDiagnose/PCBTempDiag/PCBOverTempDiag/Diagnose/Disable ==
  Action Port : ActionPort  ActionPortLabel=if(u1 == 0)
  Constant : Constant  Value=C_Flt_NoErr_b
  PCBOverTempFltDeb : Outport
  wires:
  Constant/1 -> PCBOverTempFltDeb/1

== system FaultCheck/FaultDiagnose/PCBTempDiag/PCBOverTempDiag/Diagnose/NormalDiag ==
  PCBTemp : Inport
  Parameter : Inport  Port=2
  Action Port : ActionPort  ActionPortLabel=else
  Bus Selector : BusSelector  OutputSignals=PCBOverTempConfirmTh,PCBOverTempRecoveryTh,PCBOverTempTrigTh,PCBOverTempRecTh
  DebounceRecInTwo : YS_UserDefined_Library/Fault/DebounceRecInTwo  SystemSampleTime=-1  VariantActivationTime=update diagram  Latency=0  AutoFrameSizeCalculation=off
      settings: SourceProductName=YS
  Relational Operator : RelationalOperator  Operator=<  OutDataTypeStr=boolean  RndMeth=Simplest  InputSameDT=off
  Relational Operator1 : RelationalOperator  Operator=<  OutDataTypeStr=boolean  RndMeth=Simplest  InputSameDT=off
  Signal Copy : SignalConversion  OverrideOpt=off
  PCBOverTempFltDeb : Outport
  wires:
  Parameter/1 -> Bus Selector/1
  Bus Selector/1 -> DebounceRecInTwo/1  "<PCBOverTempConfirmTh>"
  Bus Selector/2 -> DebounceRecInTwo/2  "<PCBOverTempRecoveryTh>"
  DebounceRecInTwo/1 -> Signal Copy/1  "M_Flt_PCBOverTempFltFlgDeb_b"
  Relational Operator/1 -> DebounceRecInTwo/3  "M_Flt_PCBOverTempFltFlgUnDeb_b"
  Signal Copy/1 -> PCBOverTempFltDeb/1
  Bus Selector/3 -> Relational Operator/1  "<PCBOverTempTrigTh>"
  PCBTemp/1 -> Relational Operator1/1, Relational Operator/2
  Bus Selector/4 -> Relational Operator1/2  "<PCBOverTempRecTh>"
  Relational Operator1/1 -> DebounceRecInTwo/4  "M_Flt_PCBOverTempRecFlgUnDeb_b"

== system FaultCheck/FaultDiagnose/PCBTempDiag/PCBOverTempDiag/FaultLevelDeter/LowerOne ==
  FaultLevel : Inport
  Action Port : ActionPort  ActionPortLabel=else
  PCBOverTempFltLevel : Outport
  wires:
  FaultLevel/1 -> PCBOverTempFltLevel/1

== system FaultCheck/FaultDiagnose/PCBTempDiag/PCBOverTempDiag/FaultLevelDeter/Normal ==
  Action Port : ActionPort  ActionPortLabel=if(u1 == 0)
  Constant : Constant  Value=C_Flt_LevelZero_u8
  PCBOverTempFltLevel : Outport
  wires:
  Constant/1 -> PCBOverTempFltLevel/1

== system FaultCheck/FaultDiagnose/PCBTempDiag/PCBOverTempDiag/PowerReductionCoeffDeter/If Action Subsystem ==
  Action Port : ActionPort  ActionPortLabel=if(u1 < 2)
  Constant : Constant  Value=C_Flt_PowerCoeffOne_s32
  Coeff : Outport
  wires:
  Constant/1 -> Coeff/1

== system FaultCheck/FaultDiagnose/PCBTempDiag/PCBOverTempDiag/PowerReductionCoeffDeter/If Action Subsystem1 ==
  PowerCoeff : Inport
  Action Port : ActionPort  ActionPortLabel=elseif(u1 == 2)
  Coeff : Outport
  wires:
  PowerCoeff/1 -> Coeff/1

== system FaultCheck/FaultDiagnose/PCBTempDiag/PCBOverTempDiag/PowerReductionCoeffDeter/If Action Subsystem2 ==
  Action Port : ActionPort  ActionPortLabel=else
  Constant : Constant  Value=C_Flt_PowerCoeffZero_s32
  Coeff : Outport
  wires:
  Constant/1 -> Coeff/1

== system FaultCheck/FaultDiagnose/PhaseCurrDiag/Flt_IuOverCurrDiag/Diagnose/Disable ==
  Action Port : ActionPort  ActionPortLabel=if(u1 == 0)
  Constant : Constant  Value=C_Flt_NoErr_b
  IuOCFltFlg : Outport
  wires:
  Constant/1 -> IuOCFltFlg/1

== system FaultCheck/FaultDiagnose/PhaseCurrDiag/Flt_IuOverCurrDiag/Diagnose/Enable ==
  IuOCParam : Inport
  UPhaseCurr_A : Inport  Port=2
  Action Port : ActionPort  ActionPortLabel=else
  Bus Selector : BusSelector  OutputSignals=IuOCConfirmTh,IuOCRecoveryTh,IuOCPosLimit,IuOCNegLimit
  FlgDebounce : Subsystem
  Logical Operator : Logic  AllPortsSameDT=off  OutDataTypeStr=boolean
  Relational Operator : RelationalOperator  Operator=>  OutDataTypeStr=boolean  RndMeth=Simplest  InputSameDT=off
  Relational Operator1 : RelationalOperator  Operator=<  OutDataTypeStr=boolean  RndMeth=Simplest  InputSameDT=off
  IuOCFlgDeb : Outport
  wires:
  IuOCParam/1 -> Bus Selector/1
  Bus Selector/3 -> Relational Operator1/1  "<IuOCPosLimit>"
  UPhaseCurr_A/1 -> Relational Operator/2, Relational Operator1/2
  Bus Selector/4 -> Relational Operator/1  "<IuOCNegLimit>"
  Relational Operator1/1 -> Logical Operator/1
  Relational Operator/1 -> Logical Operator/2
  Logical Operator/1 -> FlgDebounce/3(IuOCFltFlgUnDeb)  "M_Flt_IuOCFltFlgUnDeb_b"
  Bus Selector/1 -> FlgDebounce/1(ConfirmTh)  "<IuOCConfirmTh>"
  FlgDebounce/1(FlgOut) -> IuOCFlgDeb/1
  Bus Selector/2 -> FlgDebounce/2(RecoveryTh)  "<IuOCRecoveryTh>"

== system FaultCheck/FaultDiagnose/PhaseCurrDiag/Flt_IuOverCurrDiag/Diagnose/Enable Judgement ==
  SysSelfCheckDownFlg : Inport
  IuOCDiagDiagEn : Inport  Port=2
  Constant : Constant  Value=true
  Logical Operator : Logic  AllPortsSameDT=off  OutDataTypeStr=boolean
  Logical Operator1 : Logic  AllPortsSameDT=off  OutDataTypeStr=boolean
  Logical Operator2 : Logic  AllPortsSameDT=off  OutDataTypeStr=boolean
  IuOCDiagEnFlg : Outport
  wires:
  Logical Operator/1 -> IuOCDiagEnFlg/1  "M_Flt_IuOCDiagEn_b"
  Constant/1 -> Logical Operator1/1, Logical Operator2/1
  SysSelfCheckDownFlg/1 -> Logical Operator1/2
  Logical Operator2/1 -> Logical Operator/2
  Logical Operator1/1 -> Logical Operator/1
  IuOCDiagDiagEn/1 -> Logical Operator2/2

== system FaultCheck/FaultDiagnose/PhaseCurrDiag/Flt_IuOverCurrDiag/FaultLevelDeter/Normal ==
  Action Port : ActionPort  ActionPortLabel=if(u1 == 0)
  Constant : Constant  Value=C_Flt_LevelZero_u8
  IuOCFltLevel : Outport
  wires:
  Constant/1 -> IuOCFltLevel/1

== system FaultCheck/FaultDiagnose/PhaseCurrDiag/Flt_IuOverCurrDiag/FaultLevelDeter/OverCurr ==
  FaultLevel : Inport
  Action Port : ActionPort  ActionPortLabel=else
  IuOCFltLevel : Outport
  wires:
  FaultLevel/1 -> IuOCFltLevel/1

== system FaultCheck/FaultDiagnose/PhaseCurrDiag/Flt_IuOverCurrDiag/PowerReductionCoeffDeter/If Action Subsystem ==
  Action Port : ActionPort  ActionPortLabel=if(u1 < 2)
  Constant : Constant  Value=C_Flt_PowerCoeffOne_s32
  Coeff : Outport
  wires:
  Constant/1 -> Coeff/1

== system FaultCheck/FaultDiagnose/PhaseCurrDiag/Flt_IuOverCurrDiag/PowerReductionCoeffDeter/If Action Subsystem1 ==
  PowerCoeff : Inport
  Action Port : ActionPort  ActionPortLabel=elseif(u1 == 2)
  Coeff : Outport
  wires:
  PowerCoeff/1 -> Coeff/1

== system FaultCheck/FaultDiagnose/PhaseCurrDiag/Flt_IuOverCurrDiag/PowerReductionCoeffDeter/If Action Subsystem2 ==
  Action Port : ActionPort  ActionPortLabel=else
  Constant : Constant  Value=C_Flt_PowerCoeffZero_s32
  Coeff : Outport
  wires:
  Constant/1 -> Coeff/1

== system FaultCheck/FaultDiagnose/PhaseCurrDiag/Flt_IvOverCurrDiag/Diagnose/Disable ==
  Action Port : ActionPort  ActionPortLabel=if(u1 == 0)
  Constant : Constant  Value=C_Flt_NoErr_b
  IvOCFltFlg : Outport
  wires:
  Constant/1 -> IvOCFltFlg/1

== system FaultCheck/FaultDiagnose/PhaseCurrDiag/Flt_IvOverCurrDiag/Diagnose/Enable ==
  IvOCParam : Inport
  VPhaseCurr_A : Inport  Port=2
  Action Port : ActionPort  ActionPortLabel=else
  Bus Selector : BusSelector  OutputSignals=IvOCConfirmTh,IvOCRecoveryTh,IvOCPosLimit,IvOCNegLimit
  FlgDebounce : Subsystem
  Logical Operator : Logic  AllPortsSameDT=off  OutDataTypeStr=boolean
  Relational Operator : RelationalOperator  Operator=>  OutDataTypeStr=boolean  RndMeth=Simplest  InputSameDT=off
  Relational Operator1 : RelationalOperator  Operator=<  OutDataTypeStr=boolean  RndMeth=Simplest  InputSameDT=off
  IvOCFlgDeb : Outport
  wires:
  FlgDebounce/1(FlgOut) -> IvOCFlgDeb/1
  Bus Selector/1 -> FlgDebounce/1(ConfirmTh)  "<IvOCConfirmTh>"
  Logical Operator/1 -> FlgDebounce/3(IvOCFltFlgRaw)  "M_Flt_IvOCFltFlgUnDeb_b"
  Relational Operator/1 -> Logical Operator/2
  Relational Operator1/1 -> Logical Operator/1
  Bus Selector/4 -> Relational Operator/1  "<IvOCNegLimit>"
  VPhaseCurr_A/1 -> Relational Operator1/2, Relational Operator/2
  Bus Selector/3 -> Relational Operator1/1  "<IvOCPosLimit>"
  IvOCParam/1 -> Bus Selector/1
  Bus Selector/2 -> FlgDebounce/2(RecoveryTh)  "<IvOCRecoveryTh>"

== system FaultCheck/FaultDiagnose/PhaseCurrDiag/Flt_IvOverCurrDiag/Diagnose/Enable Judgement ==
  SysSelfCheckDownFlg : Inport
  IvOCDiagDiagEn : Inport  Port=2
  Constant : Constant  Value=true
  Logical Operator : Logic  AllPortsSameDT=off  OutDataTypeStr=boolean
  Logical Operator1 : Logic  AllPortsSameDT=off  OutDataTypeStr=boolean
  Logical Operator2 : Logic  AllPortsSameDT=off  OutDataTypeStr=boolean
  IvOCDiagEnFlg : Outport
  wires:
  IvOCDiagDiagEn/1 -> Logical Operator2/2
  Logical Operator1/1 -> Logical Operator/1
  Logical Operator2/1 -> Logical Operator/2
  SysSelfCheckDownFlg/1 -> Logical Operator1/2
  Constant/1 -> Logical Operator2/1, Logical Operator1/1
  Logical Operator/1 -> IvOCDiagEnFlg/1  "M_Flt_IvOCDiagEn_b"

== system FaultCheck/FaultDiagnose/PhaseCurrDiag/Flt_IvOverCurrDiag/FaultLevelDeter/Normal ==
  Action Port : ActionPort  ActionPortLabel=if(u1 == 0)
  Constant : Constant  Value=C_Flt_LevelZero_u8
  IvOCFltLevel : Outport
  wires:
  Constant/1 -> IvOCFltLevel/1

== system FaultCheck/FaultDiagnose/PhaseCurrDiag/Flt_IvOverCurrDiag/FaultLevelDeter/OverCurr ==
  FaultLevel : Inport
  Action Port : ActionPort  ActionPortLabel=else
  IvOCFltLevel : Outport
  wires:
  FaultLevel/1 -> IvOCFltLevel/1

== system FaultCheck/FaultDiagnose/PhaseCurrDiag/Flt_IvOverCurrDiag/PowerReductionCoeffDeter/If Action Subsystem ==
  Action Port : ActionPort  ActionPortLabel=if(u1 < 2)
  Constant : Constant  Value=C_Flt_PowerCoeffOne_s32
  Coeff : Outport
  wires:
  Constant/1 -> Coeff/1

== system FaultCheck/FaultDiagnose/PhaseCurrDiag/Flt_IvOverCurrDiag/PowerReductionCoeffDeter/If Action Subsystem1 ==
  PowerCoeff : Inport
  Action Port : ActionPort  ActionPortLabel=elseif(u1 == 2)
  Coeff : Outport
  wires:
  PowerCoeff/1 -> Coeff/1

== system FaultCheck/FaultDiagnose/PhaseCurrDiag/Flt_IvOverCurrDiag/PowerReductionCoeffDeter/If Action Subsystem2 ==
  Action Port : ActionPort  ActionPortLabel=else
  Constant : Constant  Value=C_Flt_PowerCoeffZero_s32
  Coeff : Outport
  wires:
  Constant/1 -> Coeff/1

== system FaultCheck/FaultDiagnose/PhaseCurrDiag/Flt_IwOverCurrDiag/Diagnose/Disable ==
  Action Port : ActionPort  ActionPortLabel=if(u1 == 0)
  Constant : Constant  Value=C_Flt_NoErr_b
  IwOCFltFlg : Outport
  wires:
  Constant/1 -> IwOCFltFlg/1

== system FaultCheck/FaultDiagnose/PhaseCurrDiag/Flt_IwOverCurrDiag/Diagnose/Enable ==
  IwOCParam : Inport
  VPhaseCurr_A : Inport  Port=2
  Action Port : ActionPort  ActionPortLabel=else
  Bus Selector : BusSelector  OutputSignals=IwOCConfirmTh,IwOCRecoveryTh,IwOCPosLimit,IwOCNegLimit
  FlgDebounce : Subsystem
  Logical Operator : Logic  AllPortsSameDT=off  OutDataTypeStr=boolean
  Relational Operator : RelationalOperator  Operator=>  OutDataTypeStr=boolean  RndMeth=Simplest  InputSameDT=off
  Relational Operator1 : RelationalOperator  Operator=<  OutDataTypeStr=boolean  RndMeth=Simplest  InputSameDT=off
  IwOCFlgDeb : Outport
  wires:
  IwOCParam/1 -> Bus Selector/1
  Bus Selector/3 -> Relational Operator1/1  "<IwOCPosLimit>"
  VPhaseCurr_A/1 -> Relational Operator/2, Relational Operator1/2
  Bus Selector/4 -> Relational Operator/1  "<IwOCNegLimit>"
  Relational Operator1/1 -> Logical Operator/1
  Relational Operator/1 -> Logical Operator/2
  Logical Operator/1 -> FlgDebounce/3(IwOCFltFlgRaw)  "M_Flt_IwOCFltFlgUnDeb_b"
  Bus Selector/1 -> FlgDebounce/1(ConfirmTh)  "<IwOCConfirmTh>"
  FlgDebounce/1(FlgOut) -> IwOCFlgDeb/1
  Bus Selector/2 -> FlgDebounce/2(RecoveryTh)  "<IwOCRecoveryTh>"

== system FaultCheck/FaultDiagnose/PhaseCurrDiag/Flt_IwOverCurrDiag/Diagnose/Enable Judgement ==
  SysSelfCheckDownFlg : Inport
  IwOCDiagDiagEn : Inport  Port=2
  Constant : Constant  Value=true
  Logical Operator : Logic  AllPortsSameDT=off  OutDataTypeStr=boolean
  Logical Operator1 : Logic  AllPortsSameDT=off  OutDataTypeStr=boolean
  Logical Operator2 : Logic  AllPortsSameDT=off  OutDataTypeStr=boolean
  IwOCDiagEnFlg : Outport
  wires:
  Logical Operator/1 -> IwOCDiagEnFlg/1  "M_Flt_IwOCDiagEn_b"
  Constant/1 -> Logical Operator1/1, Logical Operator2/1
  SysSelfCheckDownFlg/1 -> Logical Operator1/2
  Logical Operator2/1 -> Logical Operator/2
  Logical Operator1/1 -> Logical Operator/1
  IwOCDiagDiagEn/1 -> Logical Operator2/2

== system FaultCheck/FaultDiagnose/PhaseCurrDiag/Flt_IwOverCurrDiag/FaultLevelDeter/Normal ==
  Action Port : ActionPort  ActionPortLabel=if(u1 == 0)
  Constant : Constant  Value=C_Flt_LevelZero_u8
  IwOCFltLevel : Outport
  wires:
  Constant/1 -> IwOCFltLevel/1

== system FaultCheck/FaultDiagnose/PhaseCurrDiag/Flt_IwOverCurrDiag/FaultLevelDeter/OverCurr ==
  FaultLevel : Inport
  Action Port : ActionPort  ActionPortLabel=else
  IwOCFltLevel : Outport
  wires:
  FaultLevel/1 -> IwOCFltLevel/1

== system FaultCheck/FaultDiagnose/PhaseCurrDiag/Flt_IwOverCurrDiag/PowerReductionCoeffDeter/If Action Subsystem ==
  Action Port : ActionPort  ActionPortLabel=if(u1 < 2)
  Constant : Constant  Value=C_Flt_PowerCoeffOne_s32
  Coeff : Outport
  wires:
  Constant/1 -> Coeff/1

== system FaultCheck/FaultDiagnose/PhaseCurrDiag/Flt_IwOverCurrDiag/PowerReductionCoeffDeter/If Action Subsystem1 ==
  PowerCoeff : Inport
  Action Port : ActionPort  ActionPortLabel=elseif(u1 == 2)
  Coeff : Outport
  wires:
  PowerCoeff/1 -> Coeff/1

== system FaultCheck/FaultDiagnose/PhaseCurrDiag/Flt_IwOverCurrDiag/PowerReductionCoeffDeter/If Action Subsystem2 ==
  Action Port : ActionPort  ActionPortLabel=else
  Constant : Constant  Value=C_Flt_PowerCoeffZero_s32
  Coeff : Outport
  wires:
  Constant/1 -> Coeff/1
